simulink model "FamlyRStEnCtrl"  (R2018b)
settings: Solver=FixedStepDiscrete  StartTime=0.0  StopTime=10.0  FixedStep=0.01  RelTol=1e-3
undefined symbols (not defined in the file or in its folder): data, SecRwLtStFwdBkwdEn_Clear, SecRwLtStFwdBkwdEn_Set, SecRwLtStLtwdRtwdEn_Clear, SecRwLtStLtwdRtwdEn_Set, SecRwRtStFwdBkwdEn_Clear, SecRwRtStFwdBkwdEn_Set, SecRwRtStLtwdRtwdEn_Clear, SecRwRtStLtwdRtwdEn_Set, ThdRwLtStFwdBkwdEn_Clear, ThdRwLtStFwdBkwdEn_Set, ThdRwRtStFwdBkwdEn_Clear, ThdRwRtStFwdBkwdEn_Set
libraries: simulink x1
settings Model: Creator=sn2xws  LastModifiedBy=sn2xws
settings DataIOCC: SaveFormat=StructureWithTime
settings OptimizationCC: DefaultParameterBehavior=Inlined  EnhancedBackFolding=on  PassReuseOutputArgsAs=Individual arguments  ZeroExternalMemoryAtStartup=off  ZeroInternalMemoryAtStartup=off  OptimizeBlockOrder=speed  DifferentSizesBufferReuse=on  OptimizationCustomize=off
settings DebuggingCC: ParameterTunabilityLossMsg=error
settings ModelReferenceCC: ModelReferenceNumInstancesAllowed=Single
settings SFSimCC: MATLABDynamicMemAlloc=off
settings RTWCC: SystemTargetFile=autosar.tlc  GenCodeOnly=on  TemplateMakefile=ert_default_tmf  Description=AUTOSAR  GenerateReport=on  IncludeHyperlinkInReport=on  LaunchReport=on  GenerateTraceInfo=on  GenerateTraceReport=on  GenerateTraceReportSl=on  GenerateTraceReportSf=on  GenerateTraceReportEml=on  GenerateCodeMetricsReport=on
settings CodeAppCC: ForceParamTrailComments=on  IgnoreCustomStorageClasses=off  OperatorAnnotations=on  SimulinkDataObjDesc=on  SFDataObjDesc=on  InsertBlockDesc=on
settings STFCustomTargetCC: TargetLangStandard=C99 (ISO)  MultiwordLength=256  ParMdlRefBuildCompliant=on  CompOptLevelCompliant=on  IncludeMdlTerminateFcn=off  CombineOutputUpdateFcns=on  SuppressErrorStatus=on  ERTCustomFileBanners=on  SupportNonFinite=off  SupportComplex=off  SupportContinuousTime=off  SupportNonInlinedSFcns=off  RemoveResetFunc=on  MATLABClassNameForMDSCustomization=Simulink.SoftwareTarget.ERTCustomization  AutosarCompliant=on  UseToolchainInfoCompliant=on  LookupTableObjectStructAxisOrder=2,1,3,4,...  LUTObjectStructOrderEvenSpacing=Size,Table,Breakpoints  SystemTargetFile=autosar.tlc
settings ERTTargetCC: TargetLangStandard=C99 (ISO)  ConcurrentExecutionCompliant=off  IncludeMdlTerminateFcn=off  SuppressErrorStatus=on  SupportNonFinite=off  SupportComplex=off  ModelStepFunctionPrototypeControlCompliant=off  CPPClassGenCompliant=off  AutosarCompliant=on  LookupTableObjectStructAxisOrder=2,1,3,4,...  LUTObjectStructOrderEvenSpacing=Size,Table,Breakpoints  InlinedParameterPlacement=NonHierarchical  ERTCustomFileTemplate=example_file_process.tlc  ERTFilePackagingFormat=Compact

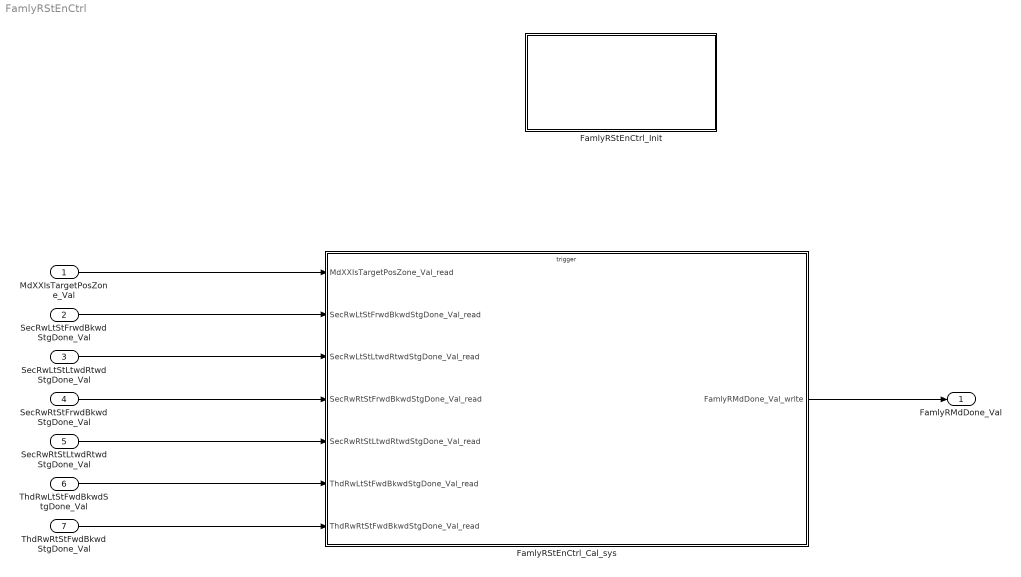
== system FamlyRStEnCtrl ==
  MdXXIsTargetPosZone_Val : Inport  OutDataTypeStr=uint32  PortDimensions=1
  SecRwLtStFrwdBkwdStgDone_Val : Inport  Port=2  OutDataTypeStr=boolean  PortDimensions=1
  SecRwLtStLtwdRtwdStgDone_Val : Inport  Port=3  OutDataTypeStr=boolean  PortDimensions=1
  SecRwRtStFrwdBkwdStgDone_Val : Inport  Port=4  OutDataTypeStr=boolean  PortDimensions=1
  SecRwRtStLtwdRtwdStgDone_Val : Inport  Port=5  OutDataTypeStr=boolean  PortDimensions=1
  ThdRwLtStFwdBkwdStgDone_Val : Inport  Port=6  OutDataTypeStr=boolean  PortDimensions=1
  ThdRwRtStFwdBkwdStgDone_Val : Inport  Port=7  OutDataTypeStr=boolean  PortDimensions=1
  FamlyRStEnCtrl_Cal_sys : Subsystem
  FamlyRStEnCtrl_Init : Subsystem
  FamlyRMdDone_Val : Outport  OutDataTypeStr=uint8  PortDimensions=1
  wires:
  MdXXIsTargetPosZone_Val/1 -> FamlyRStEnCtrl_Cal_sys/1(MdXXIsTargetPosZone_Val_read)
  SecRwLtStFrwdBkwdStgDone_Val/1 -> FamlyRStEnCtrl_Cal_sys/2(SecRwLtStFrwdBkwdStgDone_Val_read)
  SecRwLtStLtwdRtwdStgDone_Val/1 -> FamlyRStEnCtrl_Cal_sys/3(SecRwLtStLtwdRtwdStgDone_Val_read)
  SecRwRtStFrwdBkwdStgDone_Val/1 -> FamlyRStEnCtrl_Cal_sys/4(SecRwRtStFrwdBkwdStgDone_Val_read)
  SecRwRtStLtwdRtwdStgDone_Val/1 -> FamlyRStEnCtrl_Cal_sys/5(SecRwRtStLtwdRtwdStgDone_Val_read)
  ThdRwLtStFwdBkwdStgDone_Val/1 -> FamlyRStEnCtrl_Cal_sys/6(ThdRwLtStFwdBkwdStgDone_Val_read)
  ThdRwRtStFwdBkwdStgDone_Val/1 -> FamlyRStEnCtrl_Cal_sys/7(ThdRwRtStFwdBkwdStgDone_Val_read)
  FamlyRStEnCtrl_Cal_sys/1(FamlyRMdDone_Val_write) -> FamlyRMdDone_Val/1

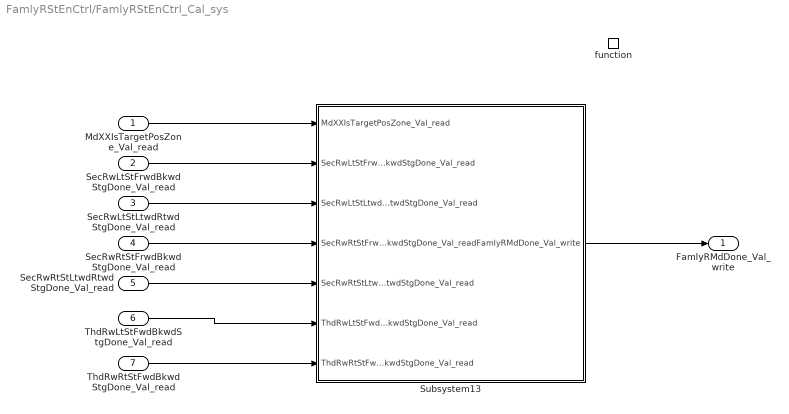
== system FamlyRStEnCtrl/FamlyRStEnCtrl_Cal_sys ==
  MdXXIsTargetPosZone_Val_read : Inport
  SecRwLtStFrwdBkwdStgDone_Val_read : Inport  Port=2
  SecRwLtStLtwdRtwdStgDone_Val_read : Inport  Port=3
  SecRwRtStFrwdBkwdStgDone_Val_read : Inport  Port=4
  SecRwRtStLtwdRtwdStgDone_Val_read : Inport  Port=5
  ThdRwLtStFwdBkwdStgDone_Val_read : Inport  Port=6
  ThdRwRtStFwdBkwdStgDone_Val_read : Inport  Port=7
  function : TriggerPort  TriggerType=function-call  IsSimulinkFunction=on  FunctionName=FamlyRStEnCtrl_Cal  VariantControl=(inherit)
  Subsystem13 : Subsystem
  FamlyRMdDone_Val_write : Outport
      settings: EnsureOutportIsVirtual=on
  wires:
  MdXXIsTargetPosZone_Val_read/1 -> Subsystem13/1(MdXXIsTargetPosZone_Val_read)
  SecRwLtStFrwdBkwdStgDone_Val_read/1 -> Subsystem13/2(SecRwLtStFrwdBkwdStgDone_Val_read)
  SecRwLtStLtwdRtwdStgDone_Val_read/1 -> Subsystem13/3(SecRwLtStLtwdRtwdStgDone_Val_read)
  SecRwRtStFrwdBkwdStgDone_Val_read/1 -> Subsystem13/4(SecRwRtStFrwdBkwdStgDone_Val_read)
  SecRwRtStLtwdRtwdStgDone_Val_read/1 -> Subsystem13/5(SecRwRtStLtwdRtwdStgDone_Val_read)
  ThdRwLtStFwdBkwdStgDone_Val_read/1 -> Subsystem13/6(ThdRwLtStFwdBkwdStgDone_Val_read)
  ThdRwRtStFwdBkwdStgDone_Val_read/1 -> Subsystem13/7(ThdRwRtStFwdBkwdStgDone_Val_read)
  Subsystem13/1(FamlyRMdDone_Val_write) -> FamlyRMdDone_Val_write/1

== system FamlyRStEnCtrl/FamlyRStEnCtrl_Init ==
  Event Listener : EventListener  EventName=reset

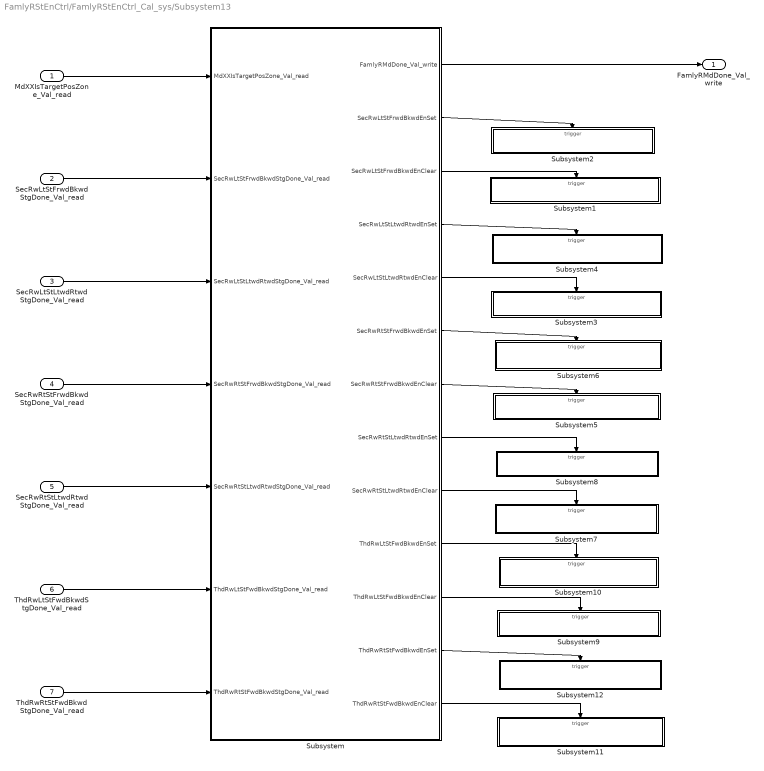
== system FamlyRStEnCtrl/FamlyRStEnCtrl_Cal_sys/Subsystem13 ==
  MdXXIsTargetPosZone_Val_read : Inport
  SecRwLtStFrwdBkwdStgDone_Val_read : Inport  Port=2
  SecRwLtStLtwdRtwdStgDone_Val_read : Inport  Port=3
  SecRwRtStFrwdBkwdStgDone_Val_read : Inport  Port=4
  SecRwRtStLtwdRtwdStgDone_Val_read : Inport  Port=5
  ThdRwLtStFwdBkwdStgDone_Val_read : Inport  Port=6
  ThdRwRtStFwdBkwdStgDone_Val_read : Inport  Port=7
  Subsystem : Subsystem
  Subsystem1 : Subsystem
  Subsystem10 : Subsystem
  Subsystem11 : Subsystem
  Subsystem12 : Subsystem
  Subsystem2 : Subsystem
  Subsystem3 : Subsystem
  Subsystem4 : Subsystem
  Subsystem5 : Subsystem
  Subsystem6 : Subsystem
  Subsystem7 : Subsystem
  Subsystem8 : Subsystem
  Subsystem9 : Subsystem
  FamlyRMdDone_Val_write : Outport
      settings: EnsureOutportIsVirtual=on
  wires:
  Subsystem/8(SecRwRtStLtwdRtwdEnSet) -> Subsystem8/Trigger
  Subsystem/2(SecRwLtStFrwdBkwdEnSet) -> Subsystem2/Trigger
  SecRwLtStLtwdRtwdStgDone_Val_read/1 -> Subsystem/3(SecRwLtStLtwdRtwdStgDone_Val_read)
  ThdRwLtStFwdBkwdStgDone_Val_read/1 -> Subsystem/6(ThdRwLtStFwdBkwdStgDone_Val_read)
  MdXXIsTargetPosZone_Val_read/1 -> Subsystem/1(MdXXIsTargetPosZone_Val_read)
  SecRwLtStFrwdBkwdStgDone_Val_read/1 -> Subsystem/2(SecRwLtStFrwdBkwdStgDone_Val_read)
  Subsystem/4(SecRwLtStLtwdRtwdEnSet) -> Subsystem4/Trigger
  Subsystem/5(SecRwLtStLtwdRtwdEnClear) -> Subsystem3/Trigger
  SecRwRtStLtwdRtwdStgDone_Val_read/1 -> Subsystem/5(SecRwRtStLtwdRtwdStgDone_Val_read)
  SecRwRtStFrwdBkwdStgDone_Val_read/1 -> Subsystem/4(SecRwRtStFrwdBkwdStgDone_Val_read)
  Subsystem/1(FamlyRMdDone_Val_write) -> FamlyRMdDone_Val_write/1
  Subsystem/12(ThdRwRtStFwdBkwdEnSet) -> Subsystem12/Trigger
  ThdRwRtStFwdBkwdStgDone_Val_read/1 -> Subsystem/7(ThdRwRtStFwdBkwdStgDone_Val_read)
  Subsystem/7(SecRwRtStFrwdBkwdEnClear) -> Subsystem5/Trigger
  Subsystem/9(SecRwRtStLtwdRtwdEnClear) -> Subsystem7/Trigger
  Subsystem/10(ThdRwLtStFwdBkwdEnSet) -> Subsystem10/Trigger
  Subsystem/3(SecRwLtStFrwdBkwdEnClear) -> Subsystem1/Trigger
  Subsystem/6(SecRwRtStFrwdBkwdEnSet) -> Subsystem6/Trigger
  Subsystem/13(ThdRwRtStFwdBkwdEnClear) -> Subsystem11/Trigger
  Subsystem/11(ThdRwLtStFwdBkwdEnClear) -> Subsystem9/Trigger

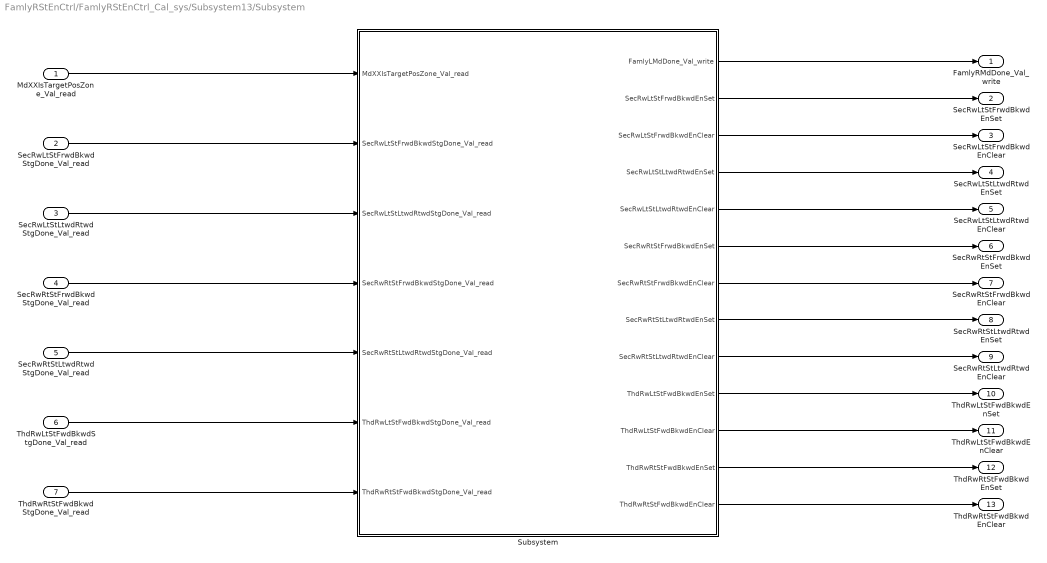
== system FamlyRStEnCtrl/FamlyRStEnCtrl_Cal_sys/Subsystem13/Subsystem ==
  MdXXIsTargetPosZone_Val_read : Inport
  SecRwLtStFrwdBkwdStgDone_Val_read : Inport  Port=2
  SecRwLtStLtwdRtwdStgDone_Val_read : Inport  Port=3
  SecRwRtStFrwdBkwdStgDone_Val_read : Inport  Port=4
  SecRwRtStLtwdRtwdStgDone_Val_read : Inport  Port=5
  ThdRwLtStFwdBkwdStgDone_Val_read : Inport  Port=6
  ThdRwRtStFwdBkwdStgDone_Val_read : Inport  Port=7
  Subsystem : Subsystem
  FamlyRMdDone_Val_write : Outport
      settings: EnsureOutportIsVirtual=on
  SecRwLtStFrwdBkwdEnSet : Outport  Port=2
  SecRwLtStFrwdBkwdEnClear : Outport  Port=3
  SecRwLtStLtwdRtwdEnSet : Outport  Port=4
  SecRwLtStLtwdRtwdEnClear : Outport  Port=5
  SecRwRtStFrwdBkwdEnSet : Outport  Port=6
  SecRwRtStFrwdBkwdEnClear : Outport  Port=7
  SecRwRtStLtwdRtwdEnSet : Outport  Port=8
  SecRwRtStLtwdRtwdEnClear : Outport  Port=9
  ThdRwLtStFwdBkwdEnSet : Outport  Port=10
  ThdRwLtStFwdBkwdEnClear : Outport  Port=11
  ThdRwRtStFwdBkwdEnSet : Outport  Port=12
  ThdRwRtStFwdBkwdEnClear : Outport  Port=13
  wires:
  Subsystem/1(FamlyLMdDone_Val_write) -> FamlyRMdDone_Val_write/1
  SecRwLtStFrwdBkwdStgDone_Val_read/1 -> Subsystem/2(SecRwLtStFrwdBkwdStgDone_Val_read)
  MdXXIsTargetPosZone_Val_read/1 -> Subsystem/1(MdXXIsTargetPosZone_Val_read)
  SecRwLtStLtwdRtwdStgDone_Val_read/1 -> Subsystem/3(SecRwLtStLtwdRtwdStgDone_Val_read)
  SecRwRtStFrwdBkwdStgDone_Val_read/1 -> Subsystem/4(SecRwRtStFrwdBkwdStgDone_Val_read)
  SecRwRtStLtwdRtwdStgDone_Val_read/1 -> Subsystem/5(SecRwRtStLtwdRtwdStgDone_Val_read)
  ThdRwLtStFwdBkwdStgDone_Val_read/1 -> Subsystem/6(ThdRwLtStFwdBkwdStgDone_Val_read)
  ThdRwRtStFwdBkwdStgDone_Val_read/1 -> Subsystem/7(ThdRwRtStFwdBkwdStgDone_Val_read)
  Subsystem/12(ThdRwRtStFwdBkwdEnSet) -> ThdRwRtStFwdBkwdEnSet/1
  Subsystem/2(SecRwLtStFrwdBkwdEnSet) -> SecRwLtStFrwdBkwdEnSet/1
  Subsystem/13(ThdRwRtStFwdBkwdEnClear) -> ThdRwRtStFwdBkwdEnClear/1
  Subsystem/5(SecRwLtStLtwdRtwdEnClear) -> SecRwLtStLtwdRtwdEnClear/1
  Subsystem/11(ThdRwLtStFwdBkwdEnClear) -> ThdRwLtStFwdBkwdEnClear/1
  Subsystem/3(SecRwLtStFrwdBkwdEnClear) -> SecRwLtStFrwdBkwdEnClear/1
  Subsystem/6(SecRwRtStFrwdBkwdEnSet) -> SecRwRtStFrwdBkwdEnSet/1
  Subsystem/8(SecRwRtStLtwdRtwdEnSet) -> SecRwRtStLtwdRtwdEnSet/1
  Subsystem/4(SecRwLtStLtwdRtwdEnSet) -> SecRwLtStLtwdRtwdEnSet/1
  Subsystem/9(SecRwRtStLtwdRtwdEnClear) -> SecRwRtStLtwdRtwdEnClear/1
  Subsystem/10(ThdRwLtStFwdBkwdEnSet) -> ThdRwLtStFwdBkwdEnSet/1
  Subsystem/7(SecRwRtStFrwdBkwdEnClear) -> SecRwRtStFrwdBkwdEnClear/1

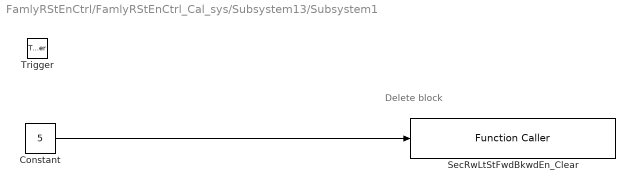
== system FamlyRStEnCtrl/FamlyRStEnCtrl_Cal_sys/Subsystem13/Subsystem1 ==
  note: Delete block
  Trigger : TriggerPort  TriggerType=function-call  VariantControl=Variant  PortDimensions=1
  Constant : Constant  Value=5  OutDataTypeStr=uint8
  SecRwLtStFwdBkwdEn_Clear : FunctionCaller  FunctionPrototype=SecRwLtStFwdBkwdEn_Clear(data)  InputArgumentSpecifications=uint8(1)
  wires:
  Constant/1 -> SecRwLtStFwdBkwdEn_Clear/1

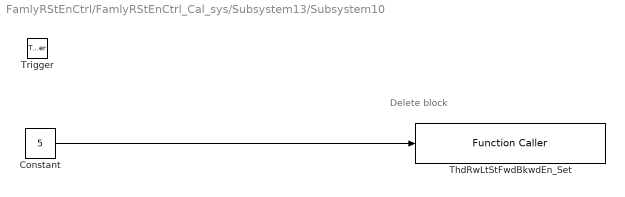
== system FamlyRStEnCtrl/FamlyRStEnCtrl_Cal_sys/Subsystem13/Subsystem10 ==
  note: Delete block
  Trigger : TriggerPort  TriggerType=function-call  VariantControl=Variant  PortDimensions=1
  Constant : Constant  Value=5  OutDataTypeStr=uint8
  ThdRwLtStFwdBkwdEn_Set : FunctionCaller  FunctionPrototype=ThdRwLtStFwdBkwdEn_Set(data)  InputArgumentSpecifications=uint8(1)
  wires:
  Constant/1 -> ThdRwLtStFwdBkwdEn_Set/1

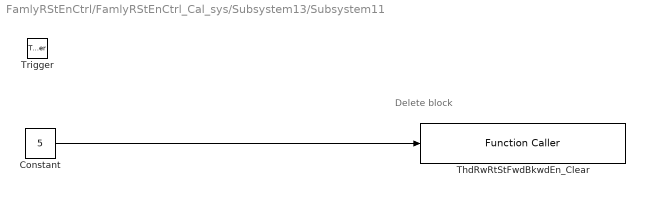
== system FamlyRStEnCtrl/FamlyRStEnCtrl_Cal_sys/Subsystem13/Subsystem11 ==
  note: Delete block
  Trigger : TriggerPort  TriggerType=function-call  VariantControl=Variant  PortDimensions=1
  Constant : Constant  Value=5  OutDataTypeStr=uint8
  ThdRwRtStFwdBkwdEn_Clear : FunctionCaller  FunctionPrototype=ThdRwRtStFwdBkwdEn_Clear(data)  InputArgumentSpecifications=uint8(1)
  wires:
  Constant/1 -> ThdRwRtStFwdBkwdEn_Clear/1

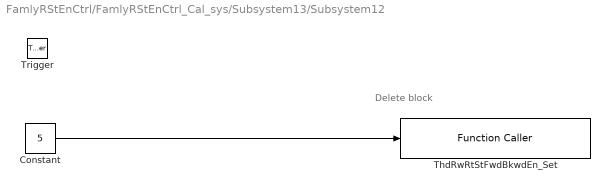
== system FamlyRStEnCtrl/FamlyRStEnCtrl_Cal_sys/Subsystem13/Subsystem12 ==
  note: Delete block
  Trigger : TriggerPort  TriggerType=function-call  VariantControl=Variant  PortDimensions=1
  Constant : Constant  Value=5  OutDataTypeStr=uint8
  ThdRwRtStFwdBkwdEn_Set : FunctionCaller  FunctionPrototype=ThdRwRtStFwdBkwdEn_Set(data)  InputArgumentSpecifications=uint8(1)
  wires:
  Constant/1 -> ThdRwRtStFwdBkwdEn_Set/1

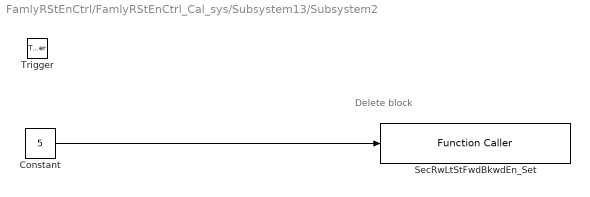
== system FamlyRStEnCtrl/FamlyRStEnCtrl_Cal_sys/Subsystem13/Subsystem2 ==
  note: Delete block
  Trigger : TriggerPort  TriggerType=function-call  VariantControl=Variant  PortDimensions=1
  Constant : Constant  Value=5  OutDataTypeStr=uint8
  SecRwLtStFwdBkwdEn_Set : FunctionCaller  FunctionPrototype=SecRwLtStFwdBkwdEn_Set(data)  InputArgumentSpecifications=uint8(1)
  wires:
  Constant/1 -> SecRwLtStFwdBkwdEn_Set/1

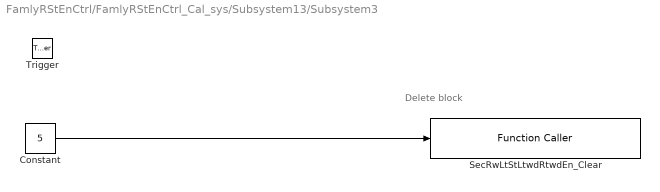
== system FamlyRStEnCtrl/FamlyRStEnCtrl_Cal_sys/Subsystem13/Subsystem3 ==
  note: Delete block
  Trigger : TriggerPort  TriggerType=function-call  VariantControl=Variant  PortDimensions=1
  Constant : Constant  Value=5  OutDataTypeStr=uint8
  SecRwLtStLtwdRtwdEn_Clear : FunctionCaller  FunctionPrototype=SecRwLtStLtwdRtwdEn_Clear(data)  InputArgumentSpecifications=uint8(1)
  wires:
  Constant/1 -> SecRwLtStLtwdRtwdEn_Clear/1

== system FamlyRStEnCtrl/FamlyRStEnCtrl_Cal_sys/Subsystem13/Subsystem4 ==
  note: Delete block
  Trigger : TriggerPort  TriggerType=function-call  VariantControl=Variant  PortDimensions=1
  Constant : Constant  Value=5  OutDataTypeStr=uint8
  SecRwLtStLtwdRtwdEn_Set : FunctionCaller  FunctionPrototype=SecRwLtStLtwdRtwdEn_Set(data)  InputArgumentSpecifications=uint8(1)
  wires:
  Constant/1 -> SecRwLtStLtwdRtwdEn_Set/1

== system FamlyRStEnCtrl/FamlyRStEnCtrl_Cal_sys/Subsystem13/Subsystem5 ==
  note: Delete block
  Trigger : TriggerPort  TriggerType=function-call  VariantControl=Variant  PortDimensions=1
  Constant : Constant  Value=5  OutDataTypeStr=uint8
  SecRwRtStFwdBkwdEn_Clear : FunctionCaller  FunctionPrototype=SecRwRtStFwdBkwdEn_Clear(data)  InputArgumentSpecifications=uint8(1)
  wires:
  Constant/1 -> SecRwRtStFwdBkwdEn_Clear/1

== system FamlyRStEnCtrl/FamlyRStEnCtrl_Cal_sys/Subsystem13/Subsystem6 ==
  note: Delete block
  Trigger : TriggerPort  TriggerType=function-call  VariantControl=Variant  PortDimensions=1
  Constant : Constant  Value=5  OutDataTypeStr=uint8
  SecRwRtStFwdBkwdEn_Set : FunctionCaller  FunctionPrototype=SecRwRtStFwdBkwdEn_Set(data)  InputArgumentSpecifications=uint8(1)
  wires:
  Constant/1 -> SecRwRtStFwdBkwdEn_Set/1

== system FamlyRStEnCtrl/FamlyRStEnCtrl_Cal_sys/Subsystem13/Subsystem7 ==
  note: Delete block
  Trigger : TriggerPort  TriggerType=function-call  VariantControl=Variant  PortDimensions=1
  Constant : Constant  Value=5  OutDataTypeStr=uint8
  SecRwRtStLtwdRtwdEn_Clear : FunctionCaller  FunctionPrototype=SecRwRtStLtwdRtwdEn_Clear(data)  InputArgumentSpecifications=uint8(1)
  wires:
  Constant/1 -> SecRwRtStLtwdRtwdEn_Clear/1

== system FamlyRStEnCtrl/FamlyRStEnCtrl_Cal_sys/Subsystem13/Subsystem8 ==
  note: Delete block
  Trigger : TriggerPort  TriggerType=function-call  VariantControl=Variant  PortDimensions=1
  Constant : Constant  Value=5  OutDataTypeStr=uint8
  SecRwRtStLtwdRtwdEn_Set : FunctionCaller  FunctionPrototype=SecRwRtStLtwdRtwdEn_Set(data)  InputArgumentSpecifications=uint8(1)
  wires:
  Constant/1 -> SecRwRtStLtwdRtwdEn_Set/1

== system FamlyRStEnCtrl/FamlyRStEnCtrl_Cal_sys/Subsystem13/Subsystem9 ==
  note: Delete block
  Trigger : TriggerPort  TriggerType=function-call  VariantControl=Variant  PortDimensions=1
  Constant : Constant  Value=5  OutDataTypeStr=uint8
  ThdRwLtStFwdBkwdEn_Clear : FunctionCaller  FunctionPrototype=ThdRwLtStFwdBkwdEn_Clear(data)  InputArgumentSpecifications=uint8(1)
  wires:
  Constant/1 -> ThdRwLtStFwdBkwdEn_Clear/1

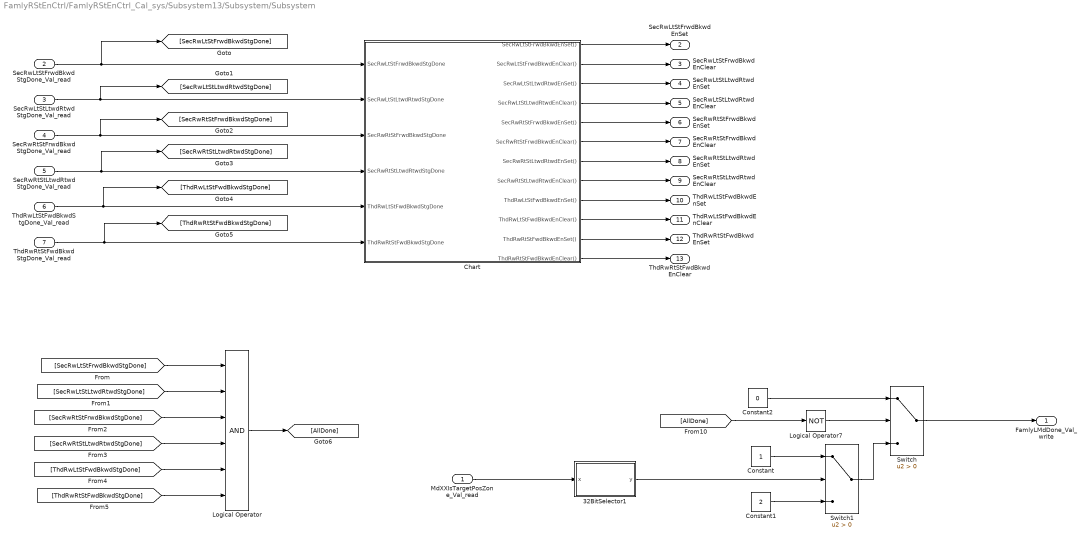
== system FamlyRStEnCtrl/FamlyRStEnCtrl_Cal_sys/Subsystem13/Subsystem/Subsystem ==
  MdXXIsTargetPosZone_Val_read : Inport
  SecRwLtStFrwdBkwdStgDone_Val_read : Inport  Port=2
  SecRwLtStLtwdRtwdStgDone_Val_read : Inport  Port=3
  SecRwRtStFrwdBkwdStgDone_Val_read : Inport  Port=4
  SecRwRtStLtwdRtwdStgDone_Val_read : Inport  Port=5
  ThdRwLtStFwdBkwdStgDone_Val_read : Inport  Port=6
  ThdRwRtStFwdBkwdStgDone_Val_read : Inport  Port=7
  32BitSelector1 : Subsystem  mask(32 Bit Selector){BitNum=5}
      mask prompts: BitNum "Select Bit Number"
      mask help: Allows selection of a particular bit (0-31) out of a packed word up to 32 bits long. Output will be true if the bit number selected via the mask parameter is equal to one.
      mask TypeOptions BitNum: 0 | 1 | 2 | 3 | 4 | 5 | 6 | 7 | 8 | 9 | 10 | 11 | 12 | 13 | 14 | 15 | 16 | 17 | 18 | 19 | 20 | 21 | 22 | 23 | 24 | 25 | 26 | 27 | 28 | 29 | 30 | 31
      mask Display:
      | text(0.5, 0.8,'BIT','horizontalAlignment','center')
      | text(0.5, 0.5,'SELECTOR','horizontalAlignment','center')
      | text(0.5, 0.2,['-- Bit ',char(get_param(gcb,'BitNum')),' --'],'horizontalAlignment','center')
  Chart : Stateflow chart  TreatAsAtomicUnit=on
  Constant : Constant  OutDataTypeStr=uint8
  Constant1 : Constant  Value=2  OutDataTypeStr=uint8
  Constant2 : Constant  Value=0  OutDataTypeStr=uint8
  Logical Operator : Logic  Inputs=6  AllPortsSameDT=off  OutDataTypeStr=boolean
  Logical Operator7 : Logic  Operator=NOT  AllPortsSameDT=off  OutDataTypeStr=boolean
  Switch : Switch  Criteria=u2 > Threshold
  Switch1 : Switch  Criteria=u2 > Threshold
  FamlyLMdDone_Val_write : Outport
      settings: EnsureOutportIsVirtual=on
  SecRwLtStFrwdBkwdEnSet : Outport  Port=2
  SecRwLtStFrwdBkwdEnClear : Outport  Port=3
  SecRwLtStLtwdRtwdEnSet : Outport  Port=4
  SecRwLtStLtwdRtwdEnClear : Outport  Port=5
  SecRwRtStFrwdBkwdEnSet : Outport  Port=6
  SecRwRtStFrwdBkwdEnClear : Outport  Port=7
  SecRwRtStLtwdRtwdEnSet : Outport  Port=8
  SecRwRtStLtwdRtwdEnClear : Outport  Port=9
  ThdRwLtStFwdBkwdEnSet : Outport  Port=10
  ThdRwLtStFwdBkwdEnClear : Outport  Port=11
  ThdRwRtStFwdBkwdEnSet : Outport  Port=12
  ThdRwRtStFwdBkwdEnClear : Outport  Port=13
  wires:
  MdXXIsTargetPosZone_Val_read/1 -> 32BitSelector1/1(x)
  Switch1/1 -> Switch/3
  [AllDone] -> Logical Operator7/1
  Switch/1 -> FamlyLMdDone_Val_write/1
  SecRwLtStFrwdBkwdStgDone_Val_read/1 -> [SecRwLtStFrwdBkwdStgDone], Chart/1(SecRwLtStFrwdBkwdStgDone)
  SecRwLtStLtwdRtwdStgDone_Val_read/1 -> [SecRwLtStLtwdRtwdStgDone], Chart/2(SecRwLtStLtwdRtwdStgDone)
  SecRwRtStFrwdBkwdStgDone_Val_read/1 -> [SecRwRtStFrwdBkwdStgDone], Chart/3(SecRwRtStFrwdBkwdStgDone)
  SecRwRtStLtwdRtwdStgDone_Val_read/1 -> [SecRwRtStLtwdRtwdStgDone], Chart/4(SecRwRtStLtwdRtwdStgDone)
  ThdRwLtStFwdBkwdStgDone_Val_read/1 -> [ThdRwLtStFwdBkwdStgDone], Chart/5(ThdRwLtStFwdBkwdStgDone)
  Chart/1(SecRwLtStFrwdBkwdEnSet()) -> SecRwLtStFrwdBkwdEnSet/1
  Chart/2(SecRwLtStFrwdBkwdEnClear()) -> SecRwLtStFrwdBkwdEnClear/1
  Chart/3(SecRwLtStLtwdRtwdEnSet()) -> SecRwLtStLtwdRtwdEnSet/1
  Chart/4(SecRwLtStLtwdRtwdEnClear()) -> SecRwLtStLtwdRtwdEnClear/1
  Chart/5(SecRwRtStFrwdBkwdEnSet()) -> SecRwRtStFrwdBkwdEnSet/1
  Chart/6(SecRwRtStFrwdBkwdEnClear()) -> SecRwRtStFrwdBkwdEnClear/1
  Chart/7(SecRwRtStLtwdRtwdEnSet()) -> SecRwRtStLtwdRtwdEnSet/1
  Chart/8(SecRwRtStLtwdRtwdEnClear()) -> SecRwRtStLtwdRtwdEnClear/1
  Chart/9(ThdRwLtStFwdBkwdEnSet()) -> ThdRwLtStFwdBkwdEnSet/1
  Chart/10(ThdRwLtStFwdBkwdEnClear()) -> ThdRwLtStFwdBkwdEnClear/1
  Chart/11(ThdRwRtStFwdBkwdEnSet()) -> ThdRwRtStFwdBkwdEnSet/1
  Chart/12(ThdRwRtStFwdBkwdEnClear()) -> ThdRwRtStFwdBkwdEnClear/1
  ThdRwRtStFwdBkwdStgDone_Val_read/1 -> [ThdRwRtStFwdBkwdStgDone], Chart/6(ThdRwRtStFwdBkwdStgDone)
  [ThdRwRtStFwdBkwdStgDone] -> Logical Operator/6
  [ThdRwLtStFwdBkwdStgDone] -> Logical Operator/5
  [SecRwRtStLtwdRtwdStgDone] -> Logical Operator/4
  [SecRwRtStFrwdBkwdStgDone] -> Logical Operator/3
  [SecRwLtStFrwdBkwdStgDone] -> Logical Operator/1
  [SecRwLtStLtwdRtwdStgDone] -> Logical Operator/2
  Logical Operator/1 -> [AllDone]
  Constant2/1 -> Switch/1
  Constant/1 -> Switch1/1
  Constant1/1 -> Switch1/3
  Logical Operator7/1 -> Switch/2
  32BitSelector1/1(y) -> Switch1/2

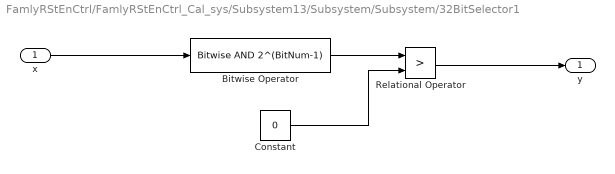
== system FamlyRStEnCtrl/FamlyRStEnCtrl_Cal_sys/Subsystem13/Subsystem/Subsystem/32BitSelector1 ==
  x : Inport
  Bitwise Operator : simulink/Logic and Bit Operations/Bitwise Operator  logicop=AND  UseBitMask=on  BitMask=2^(BitNum-1)  BitMaskRealWorld=Stored Integer
  Constant : Constant  Value=0  OutDataTypeStr=uint32
  Relational Operator : RelationalOperator  Operator=>  OutDataTypeStr=boolean  RndMeth=Simplest
  y : Outport
  wires:
  Relational Operator/1 -> y/1
  Constant/1 -> Relational Operator/2
  x/1 -> Bitwise Operator/1
  Bitwise Operator/1 -> Relational Operator/1

== stateflow chart FamlyRStEnCtrl/FamlyRStEnCtrl_Cal_sys/Subsystem13/Subsystem/Subsystem/Chart ==
  (default) -> (junction 20)
  (junction 20) -> (junction 22)
  (junction 22) -> (junction 24) [order 1] : [SecRwLtStFrwdBkwdStgDone]
  (junction 22) -> (junction 28) [order 2] : {
      | SecRwLtStFrwdBkwdEnSet;
      | }
  (junction 24) -> (junction 26) : {
      | SecRwLtStFrwdBkwdEnClear;
      | }
  (junction 26) -> (junction 28)
  (junction 28) -> (junction 39)
  (junction 39) -> (junction 31) [order 1] : [SecRwLtStLtwdRtwdStgDone]
  (junction 39) -> (junction 35) [order 2] : {
      | SecRwLtStLtwdRtwdEnSet;
      | }
  (junction 31) -> (junction 33) : {
      | SecRwLtStLtwdRtwdEnClear;
      | }
  (junction 33) -> (junction 35)
  (junction 35) -> (junction 48)
  (junction 48) -> (junction 40) [order 1] : [SecRwRtStFrwdBkwdStgDone]
  (junction 48) -> (junction 44) [order 2] : {
      | SecRwRtStFrwdBkwdEnSet;
      | }
  (junction 40) -> (junction 42) : {
      | SecRwRtStFrwdBkwdEnClear;
      | }
  (junction 42) -> (junction 44)
  (junction 44) -> (junction 57)
  (junction 57) -> (junction 49) [order 1] : [SecRwRtStLtwdRtwdStgDone]
  (junction 57) -> (junction 53) [order 2] : {
      | SecRwRtStLtwdRtwdEnSet;
      | }
  (junction 49) -> (junction 51) : {
      | SecRwRtStLtwdRtwdEnClear;
      | }
  (junction 51) -> (junction 53)
  (junction 53) -> (junction 66)
  (junction 66) -> (junction 58) [order 1] : [ThdRwLtStFwdBkwdStgDone]
  (junction 66) -> (junction 62) [order 2] : {
      | ThdRwLtStFwdBkwdEnSet;
      | }
  (junction 58) -> (junction 60) : {
      | ThdRwLtStFwdBkwdEnClear;
      | }
  (junction 60) -> (junction 62)
  (junction 62) -> (junction 75)
  (junction 75) -> (junction 67) [order 1] : [ThdRwRtStFwdBkwdStgDone]
  (junction 75) -> (junction 71) [order 2] : {
      | ThdRwRtStFwdBkwdEnSet;
      | }
  (junction 67) -> (junction 69) : {
      | ThdRwRtStFwdBkwdEnClear;
      | }
  (junction 69) -> (junction 71)
  data: SecRwLtStFrwdBkwdStgDone input boolean; SecRwLtStLtwdRtwdStgDone input boolean; SecRwRtStFrwdBkwdStgDone input boolean; SecRwRtStLtwdRtwdStgDone input boolean; ThdRwLtStFwdBkwdStgDone input boolean; ThdRwRtStFwdBkwdStgDone input boolean
  events: SecRwLtStFrwdBkwdEnSet output FUNCTION_CALL_EVENT; SecRwLtStFrwdBkwdEnClear output FUNCTION_CALL_EVENT; SecRwLtStLtwdRtwdEnSet output FUNCTION_CALL_EVENT; SecRwLtStLtwdRtwdEnClear output FUNCTION_CALL_EVENT; SecRwRtStFrwdBkwdEnSet output FUNCTION_CALL_EVENT; SecRwRtStFrwdBkwdEnClear output FUNCTION_CALL_EVENT; SecRwRtStLtwdRtwdEnSet output FUNCTION_CALL_EVENT; SecRwRtStLtwdRtwdEnClear output FUNCTION_CALL_EVENT; ThdRwLtStFwdBkwdEnSet output FUNCTION_CALL_EVENT; ThdRwLtStFwdBkwdEnClear output FUNCTION_CALL_EVENT; ThdRwRtStFwdBkwdEnSet output FUNCTION_CALL_EVENT; ThdRwRtStFwdBkwdEnClear output FUNCTION_CALL_EVENT
